simulink model "sfcndemo_sfunmem"  (Simulink 6.0)
settings: Solver=FixedStepDiscrete  StartTime=0.0  StopTime=.5  RelTol=1e-3
settings Model: Creator=The MathWorks Inc.  LastModifiedBy=batserve  ExtModeTrigMode=oneshot  ExtModeArmWhenConnect=off  ExtModeAutoUpdateStatusClock=off
settings DataIOCC: LimitDataPoints=off
settings OptimizationCC: BooleanDataType=off
settings DebuggingCC: CheckExecutionContextPreStartOutputMsg=on  CheckExecutionContextRuntimeOutputMsg=on  SolverPrmCheckMsg=none
settings HardwareCC: TargetUnknown=on

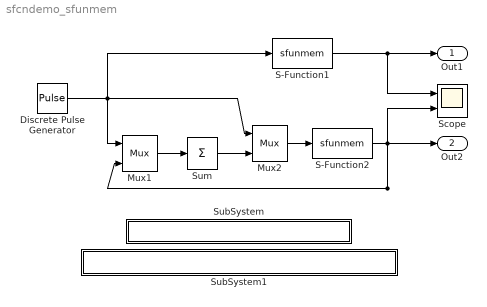
== system sfcndemo_sfunmem ==
  Discrete Pulse Generator : DiscretePulseGenerator  Period=20  PulseWidth=10  SampleTime=.01
  Mux1 : Mux  Inputs=2
  Mux2 : Mux  Inputs=2
  S-Function1 : S-Function  FunctionName=sfunmem
      mask Type: S-function: sfunmem
      mask Description: This is a S-function block which has one integration-step delay and hold "memory" function.
  S-Function2 : S-Function  FunctionName=sfunmem
      mask Type: S-function: sfunmem
      mask Description: This is a S-function block which has one integration-step delay and hold "memory" function.
  Scope : Scope  NumInputPorts=2
      settings: TimeRange=0.5  YMin=0~0  YMax=1~60
  SubSystem : Subsystem  PropExecContextAcrossSSBoundary=on
      settings: OpenFcn=edit(fullfile(matlabroot,'simulink','src','sfunmem.c'))
      mask Display: disp('matlabroot\simulink\src\sfunmem.c');
  SubSystem1 : Subsystem  PropExecContextAcrossSSBoundary=on
      settings: OpenFcn=edit(fullfile(matlabroot,'toolbox','simulink','blocks','tlc_c','sfunmem.tlc'))
      mask Display: disp('matlabroot\toolbox\simulink\blocks\tlc_c\sfunmem.tlc');
  Sum : Sum  Inputs=+  SaturateOnIntegerOverflow=on  InputSameDT=on
  Out1 : Outport
  Out2 : Outport  Port=2
  wires:
  Mux1/1 -> Sum/1
  S-Function2/1 -> Mux1/2, Scope/2, Out2/1
  Sum/1 -> Mux2/2
  Mux2/1 -> S-Function2/1
  Discrete Pulse Generator/1 -> S-Function1/1, Mux1/1, Mux2/1
  S-Function1/1 -> Out1/1, Scope/1

== system sfcndemo_sfunmem/SubSystem ==

== system sfcndemo_sfunmem/SubSystem1 ==
